simulink model "AEB_Control_2022"  (R2022b)
settings: Solver=FixedStepAuto  StartTime=0.0  StopTime=10.0  FixedStep=0.01  RelTol=1e-3
undefined symbols (not defined in the file): Distance_limit, Emgergence_Brake, Run_enable, TargetSpeed_kph
settings Model: Creator=bjkjd  LastModifiedBy=bjkjd

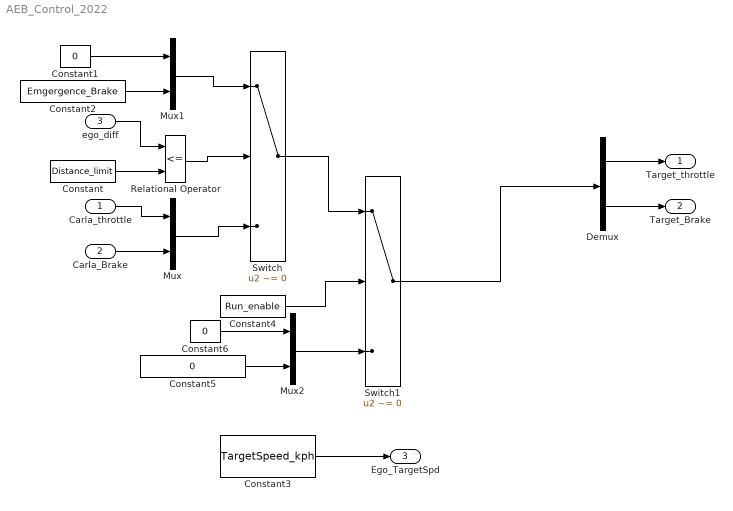
== system AEB_Control_2022 ==
  Carla_throttle : Inport  OutDataTypeStr=double
  Carla_Brake : Inport  Port=2  OutDataTypeStr=double
  ego_diff : Inport  Port=3
  Constant : Constant  Value=Distance_limit
  Constant1 : Constant  Value=0
  Constant2 : Constant  Value=Emgergence_Brake
  Constant3 : Constant  Value=TargetSpeed_kph  OutDataTypeStr=double
  Constant4 : Constant  Value=Run_enable  OutDataTypeStr=boolean
  Constant5 : Constant  Value=0
  Constant6 : Constant  Value=0
  Demux : Demux  Outputs=2
  Mux : Mux  Inputs=2
  Mux1 : Mux  Inputs=2
  Mux2 : Mux  Inputs=2
  Relational Operator : RelationalOperator  Operator=<=  OutDataTypeStr=boolean  RndMeth=Simplest  InputSameDT=off
  Switch : Switch  Criteria=u2 ~= 0  SaturateOnIntegerOverflow=off  InputSameDT=off
  Switch1 : Switch  Criteria=u2 ~= 0  SaturateOnIntegerOverflow=off  InputSameDT=off
  Target_throttle : Outport
  Target_Brake : Outport  Port=2
  Ego_TargetSpd : Outport  Port=3
  wires:
  Mux1/1 -> Switch/1
  Constant1/1 -> Mux1/1
  Constant2/1 -> Mux1/2
  ego_diff/1 -> Relational Operator/1
  Relational Operator/1 -> Switch/2
  Carla_Brake/1 -> Mux/2
  Constant/1 -> Relational Operator/2
  Carla_throttle/1 -> Mux/1
  Mux/1 -> Switch/3
  Switch1/1 -> Demux/1
  Demux/1 -> Target_throttle/1
  Demux/2 -> Target_Brake/1
  Constant3/1 -> Ego_TargetSpd/1
  Switch/1 -> Switch1/1
  Constant4/1 -> Switch1/2
  Constant5/1 -> Mux2/2
  Constant6/1 -> Mux2/1
  Mux2/1 -> Switch1/3
